simulink model "exampleStorageTnodes"  (Simulink 8.2)
settings: Solver=ode45  StartTime=0.0  StopTime=3*3600  RelTol=1e-3
undefined symbols (not defined in the file): height
libraries: carnot x17
settings Model: Creator=drhf  LastModifiedBy=drhf

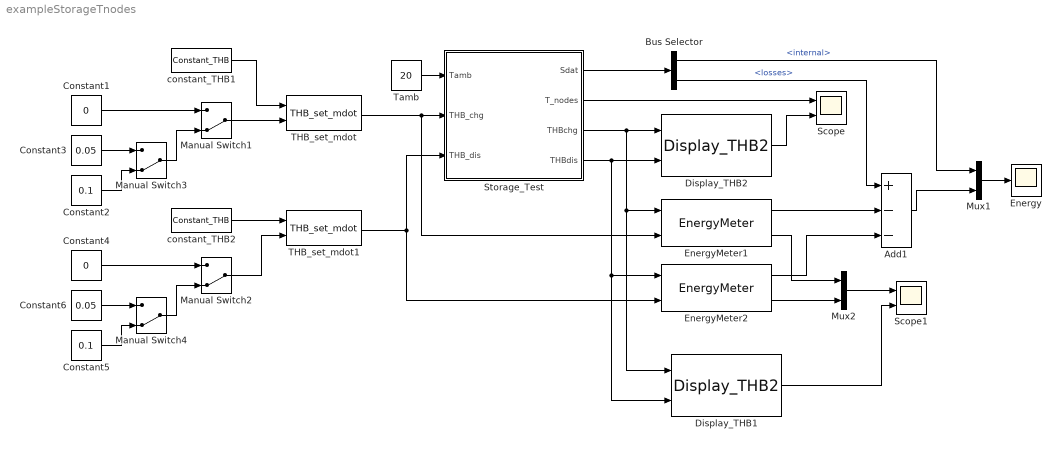
== system exampleStorageTnodes ==
  Add1 : Sum  Inputs=+--
  Bus Selector : BusSelector  OutputSignals=energy.internal,energy.losses
  Constant1 : Constant  Value=0
  Constant2 : Constant  Value=0.1
  Constant3 : Constant  Value=0.05
  Constant4 : Constant  Value=0
  Constant5 : Constant  Value=0.1
  Constant6 : Constant  Value=0.05
  Display_THB1 : carnot/Outputs/Display_THB2  t=on  m=off  p=off  id=off  mix=off  d=off
  Display_THB2 : carnot/Outputs/Display_THB2  t=off  m=on  p=off  id=off  mix=off  d=off
  Energy : Scope
  EnergyMeter1 : carnot/Control/EnergyMeter
  EnergyMeter2 : carnot/Control/EnergyMeter
  Manual Switch{1..4} (4 alike) : ManualSwitch  CurrentSetting=0
  Mux1 : Mux  Inputs=2
  Mux2 : Mux  Inputs=2
  Scope : Scope  NumInputPorts=2
      settings: YMin=-5~-5  YMax=5~5
  Scope1 : Scope  NumInputPorts=2
      settings: YMin=-5~-5  YMax=5~5  SaveName=ScopeData2
  Storage_Test : Subsystem  mask(Multiport Storage){uloss=0, ubot=0, utop=0, cond=0, t0=[10 10 55 55], volume=0.3, dia=0.5, pos=standing cylinder, nconnect=2, nodes=10, mpoints=10}
      mask prompts: uloss "Heat loss coefficient cylinder wall in W/(m²K)"; ubot "Heat loss coefficient bottom in W/(m²K)"; utop "Heat loss coefficient top cover in W/(m²K)"; cond "Effective vertical conductivity in W/(m*K)"; t0 "Initial temperature (vector or scalar) in °C"; volume "Volume in m³"; dia "Diameter in m"; pos "Position"; nconnect "Number of connections"; nodes "Number of nodes"; mpoints "Number of measurement points"
      mask help:
      | The volmue of the cylindrical storage is divided in a number "nodes" of horizontal slices (1xN-node model). For each node the energy balance equation is solved.
      | Look under mask to set the ports types and properties.
      mask init:
      | [standing, dh, height, mpts, tini] ...
      |     = CarnotCallbacks_StorageTypeN(pos, volume, dia, nodes, mpoints, t0);
      mask Help: web(fullfile(path_carnot('help'),'storage_multiport.html'),'-helpbrowser')
      mask TypeOptions pos: lying cylinder | standing cylinder
      mask Display: plot(10,10,90,100,[40,40,45,55,60,60,55,45,40],[84,36,30,30,36,84,90,90,84],[40,35],[77,77],[64,60],[77,77],[40,35],[42,42],[64,60],[42,42])
  THB_set_mdot : carnot/Source/Simple/THB_set_mdot
  THB_set_mdot1 : carnot/Source/Simple/THB_set_mdot
  Tamb : Constant  Value=20
  constant_THB1 : carnot/Source/Simple/Constant_THB  t=55  mdot=0*100/3600  p=1e5  mID=Full Pressure Drop with Static Height  fluid=Water  mix=0  dia=0.02  hgt=0
  constant_THB2 : carnot/Source/Simple/Constant_THB  t=10  mdot=100/3600  p=1e5  mID=Full Pressure Drop with Static Height  fluid=Water  mix=0  dia=0.02  hgt=0
  wires:
  Bus Selector/1 -> Mux1/1  "<internal>"
  Tamb/1 -> Storage_Test/1(Tamb)
  THB_set_mdot/1 -> EnergyMeter1/2, Storage_Test/2(THB_chg)
  THB_set_mdot1/1 -> Storage_Test/3(THB_dis), EnergyMeter2/2
  Storage_Test/1(Sdat) -> Bus Selector/1
  Storage_Test/2(T_nodes) -> Scope/1
  Storage_Test/3(THBchg) -> Display_THB2/1, EnergyMeter1/1, Display_THB1/1
  Storage_Test/4(THBdis) -> Display_THB2/2, EnergyMeter2/1, Display_THB1/2
  Display_THB2/1 -> Scope/2
  Mux1/1 -> Energy/1
  EnergyMeter2/2 -> Mux2/2
  constant_THB1/1 -> THB_set_mdot/1
  constant_THB2/1 -> THB_set_mdot1/1
  Manual Switch1/1 -> THB_set_mdot/2
  Manual Switch2/1 -> THB_set_mdot1/2
  Constant1/1 -> Manual Switch1/1
  EnergyMeter1/2 -> Mux2/1
  Add1/1 -> Mux1/2
  EnergyMeter2/1 -> Add1/3
  EnergyMeter1/1 -> Add1/2
  Bus Selector/2 -> Add1/1  "<losses>"
  Constant3/1 -> Manual Switch3/1
  Manual Switch3/1 -> Manual Switch1/2
  Constant2/1 -> Manual Switch3/2
  Constant4/1 -> Manual Switch2/1
  Constant6/1 -> Manual Switch4/1
  Manual Switch4/1 -> Manual Switch2/2
  Constant5/1 -> Manual Switch4/2
  Mux2/1 -> Scope1/1
  Display_THB1/1 -> Scope1/2

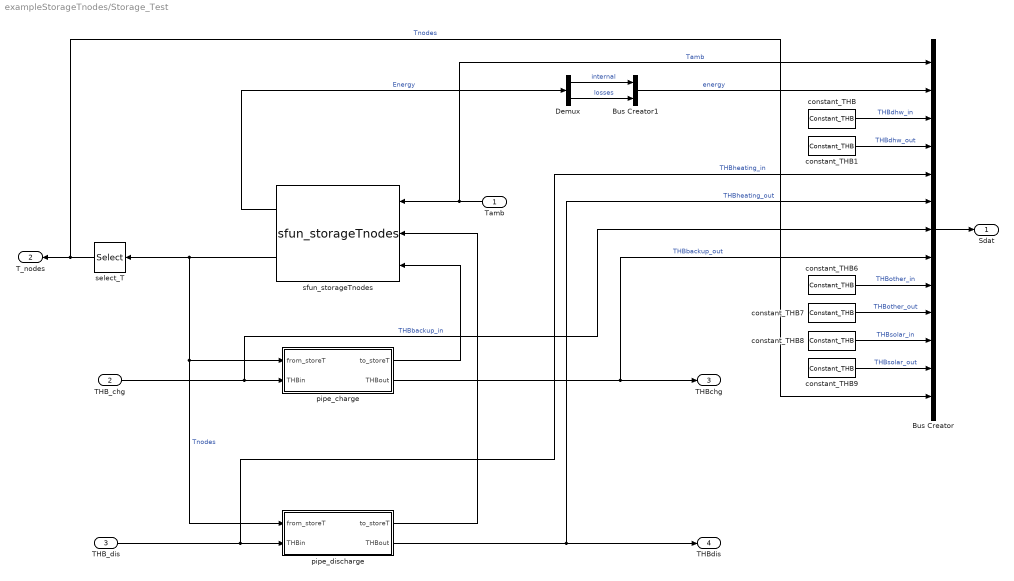
== system exampleStorageTnodes/Storage_Test ==
  Tamb : Inport
  THB_chg : Inport  Port=2
  THB_dis : Inport  Port=3
  Bus Creator : BusCreator  Inputs=13
  Bus Creator1 : BusCreator  Inputs=2
  Demux : Demux  Outputs=2
  constant_THB{,1,6..9} (6 alike) : carnot/Source/Simple/Constant_THB  t=20  mdot=0  p=1e5  mID=No Pressure Drop  fluid=Water  mix=0  dia=0.02  hgt=0
  pipe_charge : Subsystem  AncestorBlock=carnot/Storage/Thermal/Storage_Ports/Pipe  mask(pipe connection to storage){h_in=0.8, h_out=0.2, dplin=10, dpqua=10, nodes=nodes, hgt=height, dia=dia}
      mask prompts: h_in "relative height of inlet"; h_out "relative height of outlet"; dplin "linear pressure drop"; dpqua "quadratic pressure drop"; nodes "Number of nodes of storage (DO NOT CHANGE)"; hgt "Height vector (DO NOT CHANGE)"; dia "Diameter (DO NOT CHANGE)"
      mask help:
      | The block transforms the incoming THV vector to a vector which the storage interprets as a flow into the storage fluid.
      | Give inlet- and outlet-height as a relative position from 0 (= bottom) to 1 (= top).
      mask init:
      | in = zeros(nodes,1);    % vector of length nodes
      | up = in;                % vector of length nodes
      | down = in;              % vector of length nodes
      | 
      | h_in = max(0,min(h_in,1));     % no nodes below 0
      | h_out = max(0,min(h_out,1));   % no nodes below 0
      | hgt = (h_out-h_in)*hgt;
      |  
      | inlet = max(ceil(h_in*nodes),1);    % inlet position
      | outlet = max(ceil(h_out*nodes),1);  % outlet position
      |  
      | in(inlet)=1;
      |  
      | idx_in_out = inlet:outlet;
      | if (inlet < outlet)         % if inlet below outlet
      |     up(inlet:outlet-1)=1;   % upwards
      | elseif (inlet > outlet)     % else if inlet above outlet
      |     down(outlet:inlet-1)=1; % downwards
      |     idx_in_out = outlet:inlet;
      | end
      mask Help: eval('man(''pipe_connection_to_store'')')
      mask Display: disp('Pipe')
  pipe_discharge : Subsystem  AncestorBlock=carnot/Storage/Thermal/Storage_Ports/Pipe  mask(pipe connection to storage){h_in=0.2, h_out=0.8, dplin=10, dpqua=10, nodes=nodes, hgt=height, dia=dia}
      mask prompts: h_in "relative height of inlet"; h_out "relative height of outlet"; dplin "linear pressure drop"; dpqua "quadratic pressure drop"; nodes "Number of nodes of storage (DO NOT CHANGE)"; hgt "Height vector (DO NOT CHANGE)"; dia "Diameter (DO NOT CHANGE)"
      mask help:
      | The block transforms the incoming THV vector to a vector which the storage interprets as a flow into the storage fluid.
      | Give inlet- and outlet-height as a relative position from 0 (= bottom) to 1 (= top).
      mask init: same as exampleStorageTnodes/Storage_Test/pipe_charge
      mask Help: eval('man(''pipe_connection_to_store'')')
      mask Display: disp('Pipe')
  select_T : Selector  InputPortWidth=nodes  IndexOptions=Index vector (dialog)  Indices=mpts  OutputSizes=1
  sfun_storageTnodes : carnot/Basic/Thermal_Models/sfun_storageTnodes  dia=dia  volume=volume  standing=standing  uloss=uloss  ubot=utop  utop=ubot  cond=cond  tini=tini  nodes=nodes  nconnect=nconnect
  Sdat : Outport
  T_nodes : Outport  Port=2
  THBchg : Outport  Port=3
  THBdis : Outport  Port=4
  wires:
  Bus Creator1/1 -> Bus Creator/2  "energy"
  Demux/2 -> Bus Creator1/2  "losses"
  Demux/1 -> Bus Creator1/1  "internal"
  pipe_charge/1(to_storeT) -> sfun_storageTnodes/3
  pipe_charge/2(THBout) -> Bus Creator/8, THBchg/1  "THBbackup_out"
  THB_chg/1 -> Bus Creator/7, pipe_charge/2(THBin)  "THBbackup_in"
  constant_THB6/1 -> Bus Creator/9  "THBother_in"
  constant_THB7/1 -> Bus Creator/10  "THBother_out"
  constant_THB8/1 -> Bus Creator/11  "THBsolar_in"
  constant_THB9/1 -> Bus Creator/12  "THBsolar_out"
  Bus Creator/1 -> Sdat/1
  constant_THB/1 -> Bus Creator/3  "THBdhw_in"
  constant_THB1/1 -> Bus Creator/4  "THBdhw_out"
  sfun_storageTnodes/2 -> pipe_charge/1(from_storeT), pipe_discharge/1(from_storeT), select_T/1  "Tnodes"
  sfun_storageTnodes/1 -> Demux/1  "Energy"
  select_T/1 -> Bus Creator/13, T_nodes/1  "Tnodes"
  pipe_discharge/1(to_storeT) -> sfun_storageTnodes/2
  pipe_discharge/2(THBout) -> Bus Creator/6, THBdis/1  "THBheating_out"
  THB_dis/1 -> Bus Creator/5, pipe_discharge/2(THBin)  "THBheating_in"
  Tamb/1 -> sfun_storageTnodes/1, Bus Creator/1  "Tamb"

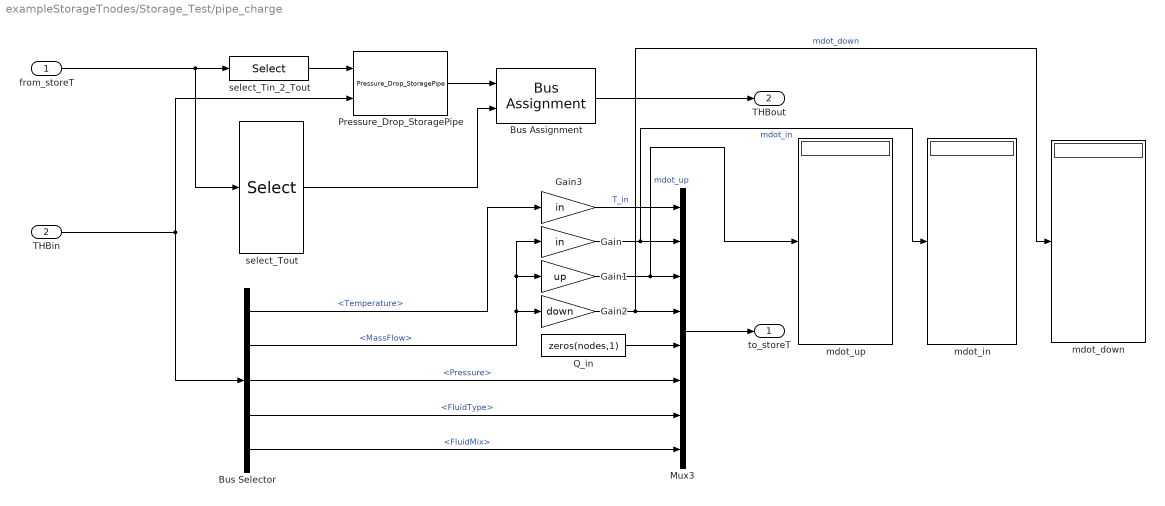
== system exampleStorageTnodes/Storage_Test/pipe_charge ==
  from_storeT : Inport
  THBin : Inport  Port=2
  Bus Assignment : BusAssignment  AssignedSignals=Temperature
  Bus Selector : BusSelector  OutputSignals=Temperature,MassFlow,Pressure,FluidType,FluidMix
  Gain : Gain  Gain=in
  Gain1 : Gain  Gain=up
  Gain2 : Gain  Gain=down
  Gain3 : Gain  Gain=in
  Mux3 : Mux  Inputs=8
  Pressure_Drop_StoragePipe : carnot/Basic/Pressure_Drop/Pressure_Drop_StoragePipe  dia=dia  hgt=hgt
  Q_in : Constant  Value=zeros(nodes,1)
  mdot_down : Display
  mdot_in : Display
  mdot_up : Display
  select_Tin_2_Tout : Selector  InputPortWidth=nodes  IndexOptions=Index vector (dialog)  Indices=[idx_in_out]  OutputSizes=1
  select_Tout : Selector  InputPortWidth=nodes  IndexOptions=Index vector (dialog)  Indices=[outlet]  OutputSizes=1
  to_storeT : Outport  InitialOutput=0
  THBout : Outport  Port=2  InitialOutput=0
  wires:
  Pressure_Drop_StoragePipe/1 -> Bus Assignment/1
  from_storeT/1 -> select_Tout/1, select_Tin_2_Tout/1
  THBin/1 -> Pressure_Drop_StoragePipe/2, Bus Selector/1
  Bus Selector/4 -> Mux3/7  "<FluidType>"
  Bus Selector/3 -> Mux3/6  "<Pressure>"
  Bus Selector/2 -> Gain/1, Gain1/1, Gain2/1  "<MassFlow>"
  Bus Selector/1 -> Gain3/1  "<Temperature>"
  Gain/1 -> Mux3/2, mdot_in/1  "mdot_in"
  Gain1/1 -> Mux3/3, mdot_up/1  "mdot_up"
  Gain2/1 -> Mux3/4, mdot_down/1  "mdot_down"
  Mux3/1 -> to_storeT/1
  select_Tout/1 -> Bus Assignment/2
  Gain3/1 -> Mux3/1  "T_in"
  Q_in/1 -> Mux3/5
  Bus Assignment/1 -> THBout/1
  Bus Selector/5 -> Mux3/8  "<FluidMix>"
  select_Tin_2_Tout/1 -> Pressure_Drop_StoragePipe/1

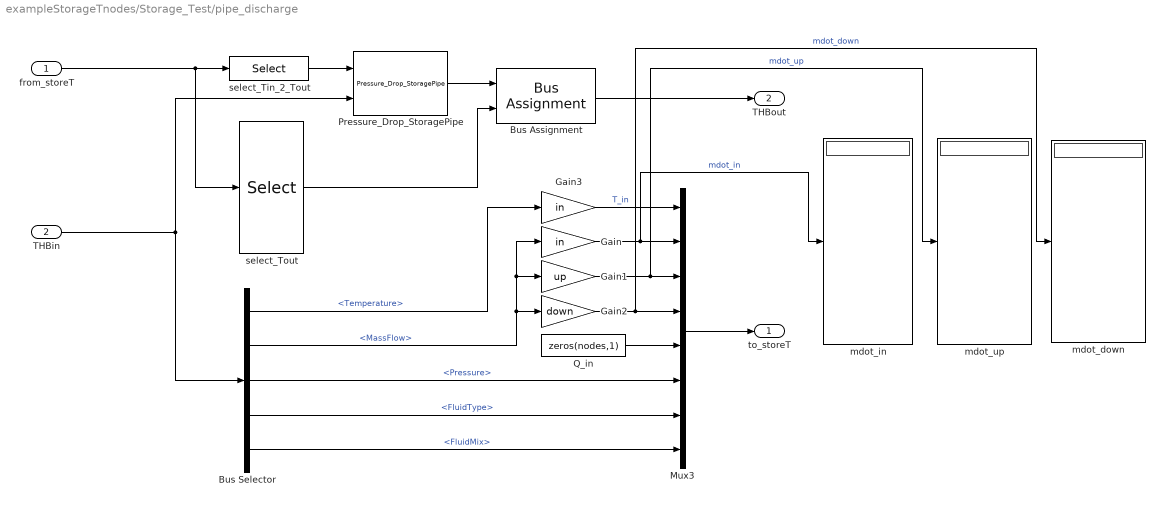
== system exampleStorageTnodes/Storage_Test/pipe_discharge ==
  from_storeT : Inport
  THBin : Inport  Port=2
  Bus Assignment : BusAssignment  AssignedSignals=Temperature
  Bus Selector : BusSelector  OutputSignals=Temperature,MassFlow,Pressure,FluidType,FluidMix
  Gain : Gain  Gain=in
  Gain1 : Gain  Gain=up
  Gain2 : Gain  Gain=down
  Gain3 : Gain  Gain=in
  Mux3 : Mux  Inputs=8
  Pressure_Drop_StoragePipe : carnot/Basic/Pressure_Drop/Pressure_Drop_StoragePipe  dia=dia  hgt=hgt
  Q_in : Constant  Value=zeros(nodes,1)
  mdot_down : Display
  mdot_in : Display
  mdot_up : Display
  select_Tin_2_Tout : Selector  InputPortWidth=nodes  IndexOptions=Index vector (dialog)  Indices=[idx_in_out]  OutputSizes=1
  select_Tout : Selector  InputPortWidth=nodes  IndexOptions=Index vector (dialog)  Indices=[outlet]  OutputSizes=1
  to_storeT : Outport  InitialOutput=0
  THBout : Outport  Port=2  InitialOutput=0
  wires:
  select_Tin_2_Tout/1 -> Pressure_Drop_StoragePipe/1
  Bus Selector/5 -> Mux3/8  "<FluidMix>"
  Bus Assignment/1 -> THBout/1
  Q_in/1 -> Mux3/5
  Gain3/1 -> Mux3/1  "T_in"
  select_Tout/1 -> Bus Assignment/2
  Mux3/1 -> to_storeT/1
  Gain2/1 -> mdot_down/1, Mux3/4  "mdot_down"
  Gain1/1 -> mdot_up/1, Mux3/3  "mdot_up"
  Gain/1 -> mdot_in/1, Mux3/2  "mdot_in"
  Bus Selector/1 -> Gain3/1  "<Temperature>"
  Bus Selector/2 -> Gain2/1, Gain1/1, Gain/1  "<MassFlow>"
  Bus Selector/3 -> Mux3/6  "<Pressure>"
  Bus Selector/4 -> Mux3/7  "<FluidType>"
  THBin/1 -> Bus Selector/1, Pressure_Drop_StoragePipe/2
  from_storeT/1 -> select_Tin_2_Tout/1, select_Tout/1
  Pressure_Drop_StoragePipe/1 -> Bus Assignment/1
